simulink model "linear_model_GFM"  (R2018b)
settings: Solver=VariableStepAuto  StartTime=0.0  StopTime=0  RelTol=1e-3
InitFcn:
  | GFM_init
values from neighbouring files (symbols this model uses):
  Cf = Bf/w0    (= 6.36619772368e-05)    [MainTest.m]    (also in MainTest_v2.m)
  L = 1/Wbase    (= 0.00318309886184)    [Test.m]
  Pr = sym('Pr')    [MainTest.m]    (also in MainTest_v2.m)
  Qr = sym('Qr')    [MainTest.m]    (also in MainTest_v2.m)
  R = 1    [Test.m]
  Tm = 50*1e-3    (= 0.05)    [MainTest.m]    (also in MainTest_v2.m)
  w0 = 50*2*pi    (= 314.159265359)    [MainTest.m]    (also in MainTest_v2.m)
undefined symbols (not defined in the file or in its folder): Dp, Dq, I_d, I_LD, I_LQ, I_q, Ki, Kp, Tc, th, V, V_d, V_q, Vs
libraries: simulink x2
settings Model: Creator=balarko  LastModifiedBy=balarko
settings DataIOCC: ReturnWorkspaceOutputs=on

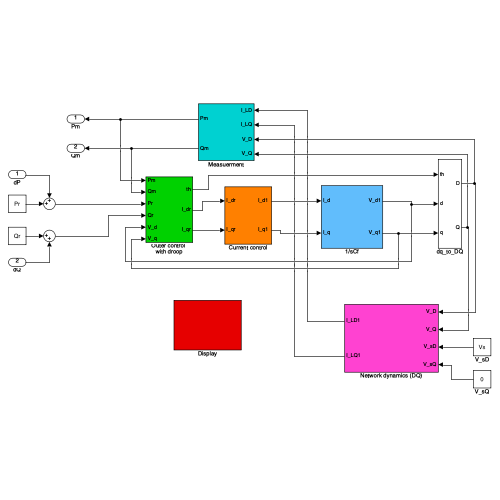
[thumbnail: Simulink's stored preview of the top-level diagram]
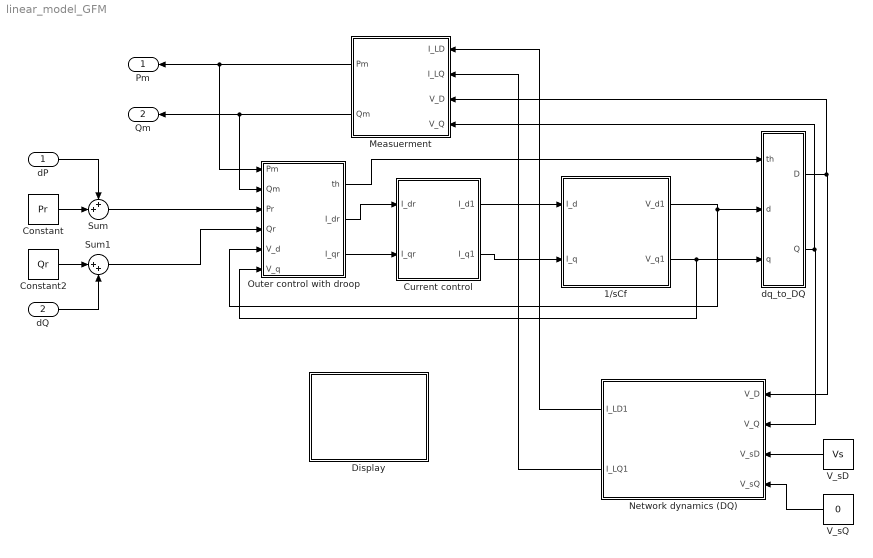
== system linear_model_GFM ==
  dP : Inport
  dQ : Inport  Port=2
  1/sCf : Subsystem
  Constant : Constant  Value=Pr
  Constant2 : Constant  Value=Qr
  Current control : Subsystem
  Display : Subsystem
  Measuerment : Subsystem
  Network dynamics (DQ) : Subsystem
  Outer control with droop : Subsystem
  Sum : Sum  Inputs=++|
  Sum1 : Sum  Inputs=|++
  V_sD : Constant  Value=Vs
  V_sQ : Constant  Value=0
  dq_to_DQ : Subsystem
  Pm : Outport
  Qm : Outport  Port=2
  wires:
  Outer control with droop/2(I_dr) -> Current control/1(I_dr)
  Outer control with droop/3(I_qr) -> Current control/2(I_qr)
  Current control/1("I_d1 ") -> 1/sCf/1(I_d)
  Current control/2("I_q1 ") -> 1/sCf/2(I_q)
  Network dynamics (DQ)/2(I_LQ1) -> Measuerment/2(I_LQ)
  1/sCf/1(V_d1) -> dq_to_DQ/2(d), Outer control with droop/5(V_d)
  1/sCf/2(V_q1) -> dq_to_DQ/3(q), Outer control with droop/6(V_q)
  V_sD/1 -> Network dynamics (DQ)/3(V_sD)
  V_sQ/1 -> Network dynamics (DQ)/4(V_sQ)
  Measuerment/2(Qm) -> Qm/1, Outer control with droop/2(Qm)
  Measuerment/1(Pm) -> Pm/1, Outer control with droop/1(Pm)
  Network dynamics (DQ)/1(I_LD1) -> Measuerment/1(I_LD)
  Sum/1 -> Outer control with droop/3(Pr)
  Constant/1 -> Sum/2
  Constant2/1 -> Sum1/1
  dQ/1 -> Sum1/2
  Sum1/1 -> Outer control with droop/4(Qr)
  dP/1 -> Sum/1
  dq_to_DQ/1(D) -> Measuerment/3(V_D), Network dynamics (DQ)/1(V_D)
  dq_to_DQ/2(Q) -> Measuerment/4(V_Q), Network dynamics (DQ)/2(V_Q)
  Outer control with droop/1(th) -> dq_to_DQ/1(th)

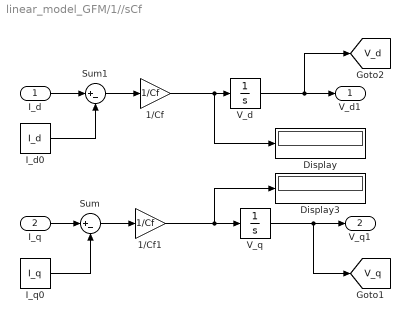
== system linear_model_GFM/1//sCf ==
  I_d : Inport
  I_q : Inport  Port=2
  1/Cf : Gain  Gain=1/Cf
  1/Cf1 : Gain  Gain=1/Cf
  Display : Display
  Display3 : Display
  I_d0 : Constant  Value=I_d
  I_q0 : Constant  Value=I_q
  Sum : Sum  Inputs=|+-
  Sum1 : Sum  Inputs=|+-
  V_d : Integrator  InitialCondition=V_d
  V_q : Integrator  InitialCondition=V_q
  V_d1 : Outport  VectorParamsAs1DForOutWhenUnconnected=off
  V_q1 : Outport  Port=2  VectorParamsAs1DForOutWhenUnconnected=off
  tag scope: V_d=global, V_q=global
  wires:
  V_d/1 -> [V_d], V_d1/1
  V_q/1 -> [V_q], V_q1/1
  1/Cf/1 -> Display/1, V_d/1
  1/Cf1/1 -> Display3/1, V_q/1
  I_q/1 -> Sum/1
  I_d/1 -> Sum1/1
  Sum1/1 -> 1/Cf/1
  I_d0/1 -> Sum1/2
  I_q0/1 -> Sum/2
  Sum/1 -> 1/Cf1/1

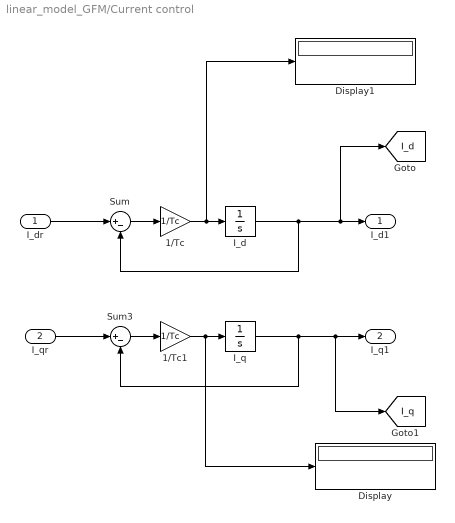
== system linear_model_GFM/Current control ==
  I_dr : Inport
  I_qr : Inport  Port=2
  1/Tc : Gain  Gain=1/Tc
  1/Tc1 : Gain  Gain=1/Tc
  Display : Display
  Display1 : Display
  "I_d " : Integrator  InitialCondition=I_d
  "I_q " : Integrator  InitialCondition=I_q
  Sum : Sum  Inputs=|+-
  Sum3 : Sum  Inputs=|+-
  "I_d1 " : Outport  VectorParamsAs1DForOutWhenUnconnected=off
  "I_q1 " : Outport  Port=2  VectorParamsAs1DForOutWhenUnconnected=off
  tag scope: I_d=global, I_q=global
  wires:
  Sum/1 -> 1/Tc/1
  1/Tc/1 -> Display1/1, "I_d "/1
  I_dr/1 -> Sum/1
  "I_d "/1 -> [I_d], "I_d1 "/1, Sum/2
  "I_q "/1 -> [I_q], "I_q1 "/1, Sum3/2
  Sum3/1 -> 1/Tc1/1
  1/Tc1/1 -> Display/1, "I_q "/1
  I_qr/1 -> Sum3/1

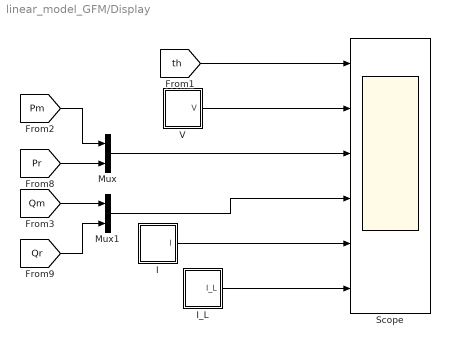
== system linear_model_GFM/Display ==
  I : Subsystem
  I_L : Subsystem
  Mux : Mux  Inputs=2
  Mux1 : Mux  Inputs=2
  Scope : Scope  NumInputPorts=6
  V : Subsystem
  wires:
  [Pr] -> Mux/2
  [Qm] -> Mux1/1
  [Qr] -> Mux1/2
  [Pm] -> Mux/1
  [th] -> Scope/1
  V/1(V) -> Scope/2
  Mux/1 -> Scope/3
  I_L/1(I_L) -> Scope/6
  I/1(I) -> Scope/5
  Mux1/1 -> Scope/4

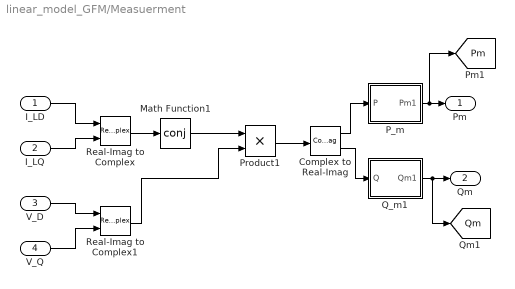
== system linear_model_GFM/Measuerment ==
  I_LD : Inport
  I_LQ : Inport  Port=2
  V_D : Inport  Port=3
  V_Q : Inport  Port=4
  Complex to Real-Imag : ComplexToRealImag
  Math Function1 : Math  Operator=conj  SaturateOnIntegerOverflow=on
  P_m : Subsystem
  Product1 : Product
  Q_m1 : Subsystem
  Real-Imag to Complex : RealImagToComplex
  Real-Imag to Complex1 : RealImagToComplex
  Pm : Outport  VectorParamsAs1DForOutWhenUnconnected=off
  Qm : Outport  Port=2  VectorParamsAs1DForOutWhenUnconnected=off
  tag scope: Pm=global, Qm=global
  wires:
  Real-Imag to Complex/1 -> Math Function1/1
  Math Function1/1 -> Product1/1
  Product1/1 -> Complex to Real-Imag/1
  Real-Imag to Complex1/1 -> Product1/2
  I_LD/1 -> Real-Imag to Complex/1
  I_LQ/1 -> Real-Imag to Complex/2
  V_D/1 -> Real-Imag to Complex1/1
  V_Q/1 -> Real-Imag to Complex1/2
  P_m/1(Pm1) -> [Pm], Pm/1
  Complex to Real-Imag/1 -> P_m/1(P)
  Complex to Real-Imag/2 -> Q_m1/1(Q)
  Q_m1/1(Qm1) -> [Qm], Qm/1

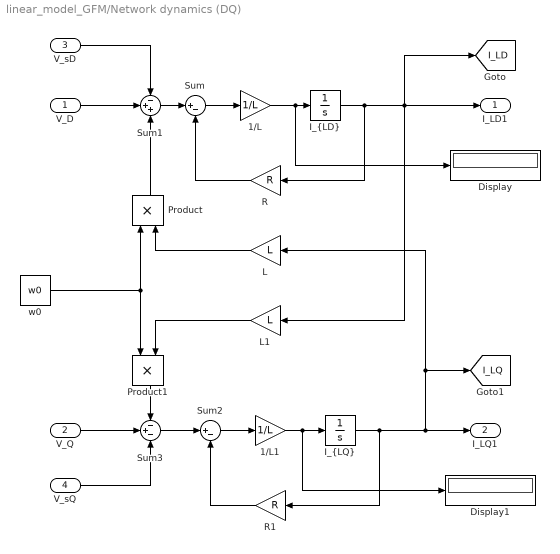
== system linear_model_GFM/Network dynamics (DQ) ==
  V_D : Inport
  V_Q : Inport  Port=2
  V_sD : Inport  Port=3
  V_sQ : Inport  Port=4
  1/L : Gain  Gain=1/L
  1/L1 : Gain  Gain=1/L
  Display : Display
  Display1 : Display
  "I_{LD}" : Integrator  InitialCondition=I_LD
  "I_{LQ}" : Integrator  InitialCondition=I_LQ
  L : Gain  Gain=L
  L1 : Gain  Gain=L
  Product : Product
  Product1 : Product
  R : Gain  Gain=R
  R1 : Gain  Gain=R
  Sum : Sum  Inputs=|+-
  Sum1 : Sum  Inputs=-++
  Sum2 : Sum  Inputs=|+-
  Sum3 : Sum  Inputs=-+-
  w0 : Constant  Value=w0
  I_LD1 : Outport  VectorParamsAs1DForOutWhenUnconnected=off
  I_LQ1 : Outport  Port=2  VectorParamsAs1DForOutWhenUnconnected=off
  tag scope: I_LD=global, I_LQ=global
  wires:
  Sum1/1 -> Sum/1
  V_sQ/1 -> Sum3/3
  1/L/1 -> Display/1, "I_{LD}"/1
  1/L1/1 -> Display1/1, "I_{LQ}"/1
  V_sD/1 -> Sum1/1
  Sum/1 -> 1/L/1
  "I_{LD}"/1 -> [I_LD], I_LD1/1, L1/1, R/1
  "I_{LQ}"/1 -> I_LQ1/1, [I_LQ], L/1, R1/1
  R/1 -> Sum/2
  Sum3/1 -> Sum2/1
  Sum2/1 -> 1/L1/1
  V_Q/1 -> Sum3/2
  R1/1 -> Sum2/2
  V_D/1 -> Sum1/2
  Product/1 -> Sum1/3
  Product1/1 -> Sum3/1
  w0/1 -> Product1/1, Product/1
  L/1 -> Product/2
  L1/1 -> Product1/2

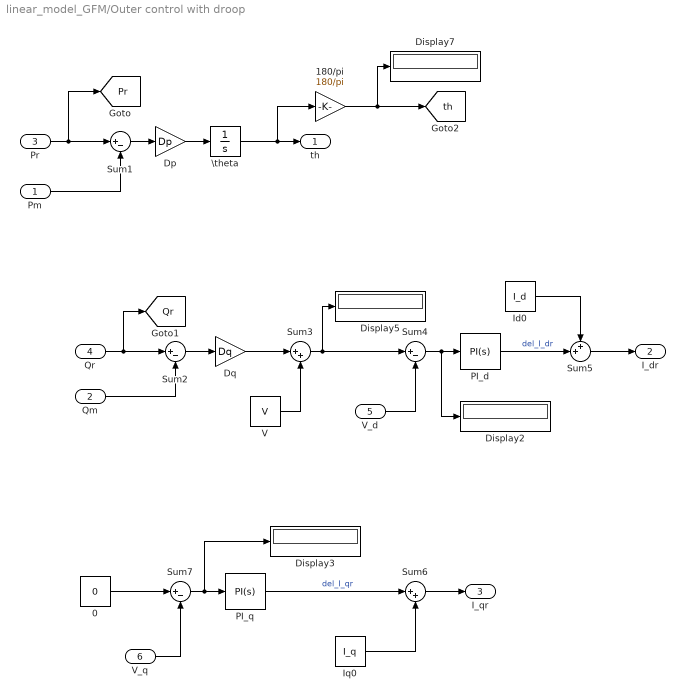
== system linear_model_GFM/Outer control with droop ==
  Pm : Inport
  Qm : Inport  Port=2
  Pr : Inport  Port=3
  Qr : Inport  Port=4
  V_d : Inport  Port=5
  V_q : Inport  Port=6
  0 : Constant  Value=0
  180/pi : Gain  Gain=180/pi
  Display{2..3,5,7} (4 alike) : Display
  Dp : Gain  Gain=Dp
  Dq : Gain  Gain=Dq
  Id0 : Constant  Value=I_d
  Iq0 : Constant  Value=I_q
  PI_d : simulink/Continuous/PID Controller  Controller=PI  Form=Parallel  TimeDomain=Continuous-time  SampleTime=-1  IntegratorMethod=Forward Euler  ControllerParametersSource=internal  P=Kp  I=Ki  D=0  N=100  UseFilter=on  TunerSelectOption=Transfer Function Based (PID Tuner App)  InitialConditionSource=internal  InitialConditionForIntegrator=0  InitialConditionForFilter=0  DifferentiatorICPrevScaledInput=0  ExternalReset=none  TrackingMode=off  Kt=1  LimitOutput=off  UpperSaturationLimit=inf  LowerSaturationLimit=-inf  LinearizeAsGain=on  AntiWindupMode=none  Kb=1  POutMin=[]  POutMax=[]  IOutMin=[]  IOutMax=[]  DOutMin=[]  DOutMax=[]  NOutMin=[]  NOutMax=[]  SumOutMin=[]  SumOutMax=[]  SaturationOutMin=[]  SaturationOutMax=[]  PParamMin=[]  PParamMax=[]  IParamMin=[]  IParamMax=[]  DParamMin=[]  DParamMax=[]  NParamMin=[]  NParamMax=[]  KbParamMin=[]  KbParamMax=[]  KtParamMin=[]  KtParamMax=[]  KbOutMin=[]  KbOutMax=[]  KtOutMin=[]  KtOutMax=[]  IntegratorOutMin=[]  IntegratorOutMax=[]  FilterOutMin=[]  FilterOutMax=[]  SumI1OutMin=[]  SumI1OutMax=[]  SumI2OutMin=[]  SumI2OutMax=[]  SumI3OutMin=[]  SumI3OutMax=[]  SumI4OutMin=[]  SumI4OutMax=[]  SumDOutMin=[]  SumDOutMax=[]  DifferentiatorOutMin=[]  DifferentiatorOutMax=[]  FilterDiffOutCoefMin=[]  FilterDiffOutCoefMax=[]  ReciprocalOutMin=[]  ReciprocalOutMax=[]  SumDenOutMin=[]  SumDenOutMax=[]  SumNumOutMin=[]  SumNumOutMax=[]  DivideOutMin=[]  DivideOutMax=[]  IntegratorContinuousStateAttributes='PI_d'  IntegratorStateMustResolveToSignalObject=off  IntegratorRTWStateStorageClass=Auto  FilterContinuousStateAttributes=''  FilterStateMustResolveToSignalObject=off  FilterRTWStateStorageClass=Auto  ParallelPVariant=InternalParameters  IdealPVariant=Disabled  IVariant=InternalParameters  DVariant=Disabled  IntegratorVariant=Continuous  SatVariant=Disabled  AWVariant=Passthrough  PCopyVariant=Disabled  TRVariant=Disabled  FdbkBlocksVariant=Forward  IdealPFdbkVariant=Disabled  SatFdbkVariant=Disabled  DerivativeFilterVariant=Disabled  NVariant=Disabled  NCopyVariant=Disabled_SignalSpec  FilterICVariant=Disabled  IntegratorICVariant=InternalICs  ExternalResetVariant=Disabled  TRSumVariant=Passthrough  SumFdbkVariant=Disabled  SumVariant=Sum_PI
  PI_q : simulink/Continuous/PID Controller  Controller=PI  Form=Parallel  TimeDomain=Continuous-time  SampleTime=-1  IntegratorMethod=Forward Euler  ControllerParametersSource=internal  P=Kp  I=Ki  D=0  N=100  UseFilter=on  TunerSelectOption=Transfer Function Based (PID Tuner App)  InitialConditionSource=internal  InitialConditionForIntegrator=0  InitialConditionForFilter=0  DifferentiatorICPrevScaledInput=0  ExternalReset=none  TrackingMode=off  Kt=1  LimitOutput=off  UpperSaturationLimit=inf  LowerSaturationLimit=-inf  LinearizeAsGain=on  AntiWindupMode=none  Kb=1  POutMin=[]  POutMax=[]  IOutMin=[]  IOutMax=[]  DOutMin=[]  DOutMax=[]  NOutMin=[]  NOutMax=[]  SumOutMin=[]  SumOutMax=[]  SaturationOutMin=[]  SaturationOutMax=[]  PParamMin=[]  PParamMax=[]  IParamMin=[]  IParamMax=[]  DParamMin=[]  DParamMax=[]  NParamMin=[]  NParamMax=[]  KbParamMin=[]  KbParamMax=[]  KtParamMin=[]  KtParamMax=[]  KbOutMin=[]  KbOutMax=[]  KtOutMin=[]  KtOutMax=[]  IntegratorOutMin=[]  IntegratorOutMax=[]  FilterOutMin=[]  FilterOutMax=[]  SumI1OutMin=[]  SumI1OutMax=[]  SumI2OutMin=[]  SumI2OutMax=[]  SumI3OutMin=[]  SumI3OutMax=[]  SumI4OutMin=[]  SumI4OutMax=[]  SumDOutMin=[]  SumDOutMax=[]  DifferentiatorOutMin=[]  DifferentiatorOutMax=[]  FilterDiffOutCoefMin=[]  FilterDiffOutCoefMax=[]  ReciprocalOutMin=[]  ReciprocalOutMax=[]  SumDenOutMin=[]  SumDenOutMax=[]  SumNumOutMin=[]  SumNumOutMax=[]  DivideOutMin=[]  DivideOutMax=[]  IntegratorContinuousStateAttributes='PI_q'  IntegratorStateMustResolveToSignalObject=off  IntegratorRTWStateStorageClass=Auto  FilterContinuousStateAttributes=''  FilterStateMustResolveToSignalObject=off  FilterRTWStateStorageClass=Auto  ParallelPVariant=InternalParameters  IdealPVariant=Disabled  IVariant=InternalParameters  DVariant=Disabled  IntegratorVariant=Continuous  SatVariant=Disabled  AWVariant=Passthrough  PCopyVariant=Disabled  TRVariant=Disabled  FdbkBlocksVariant=Forward  IdealPFdbkVariant=Disabled  SatFdbkVariant=Disabled  DerivativeFilterVariant=Disabled  NVariant=Disabled  NCopyVariant=Disabled_SignalSpec  FilterICVariant=Disabled  IntegratorICVariant=InternalICs  ExternalResetVariant=Disabled  TRSumVariant=Passthrough  SumFdbkVariant=Disabled  SumVariant=Sum_PI
  Sum{1..2,4,7} (4 alike) : Sum  Inputs=|+-
  Sum3 : Sum  Inputs=|++
  Sum5 : Sum  Inputs=++|
  Sum6 : Sum  Inputs=|++
  V : Constant  Value=V
  \theta : Integrator  InitialCondition=th*pi/180
  th : Outport
  I_dr : Outport  Port=2  VectorParamsAs1DForOutWhenUnconnected=off
  I_qr : Outport  Port=3  VectorParamsAs1DForOutWhenUnconnected=off
  tag scope: Pr=global, Qr=global, th=global
  wires:
  Pr/1 -> [Pr], Sum1/1
  Qm/1 -> Sum2/2
  Qr/1 -> [Qr], Sum2/1
  Pm/1 -> Sum1/2
  Sum1/1 -> Dp/1
  Sum2/1 -> Dq/1
  V/1 -> Sum3/2
  Sum4/1 -> Display2/1, PI_d/1
  Sum7/1 -> Display3/1, PI_q/1
  \theta/1 -> th/1, 180/pi/1
  Sum3/1 -> Sum4/1, Display5/1
  0/1 -> Sum7/1
  V_d/1 -> Sum4/2
  V_q/1 -> Sum7/2
  180/pi/1 -> Display7/1, [th]
  PI_d/1 -> Sum5/2  "del_I_dr"
  Sum5/1 -> I_dr/1
  PI_q/1 -> Sum6/1  "del_I_qr"
  Iq0/1 -> Sum6/2
  Id0/1 -> Sum5/1
  Sum6/1 -> I_qr/1
  Dp/1 -> \theta/1
  Dq/1 -> Sum3/1

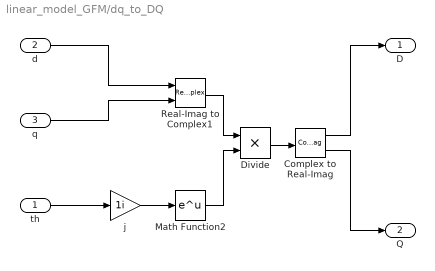
== system linear_model_GFM/dq_to_DQ ==
  th : Inport
  d : Inport  Port=2
  q : Inport  Port=3
  Complex to Real-Imag : ComplexToRealImag
  Divide : Product  Inputs=**
  Math Function2 : Math  SaturateOnIntegerOverflow=on
  Real-Imag to Complex1 : RealImagToComplex
  j : Gain  Gain=1i
  D : Outport  VectorParamsAs1DForOutWhenUnconnected=off
  Q : Outport  Port=2  VectorParamsAs1DForOutWhenUnconnected=off
  wires:
  Real-Imag to Complex1/1 -> Divide/1
  Complex to Real-Imag/2 -> Q/1
  j/1 -> Math Function2/1
  Math Function2/1 -> Divide/2
  d/1 -> Real-Imag to Complex1/1
  Complex to Real-Imag/1 -> D/1
  q/1 -> Real-Imag to Complex1/2
  Divide/1 -> Complex to Real-Imag/1
  th/1 -> j/1

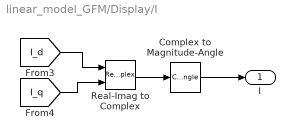
== system linear_model_GFM/Display/I ==
  Complex to Magnitude-Angle : ComplexToMagnitudeAngle  Output=Magnitude
  Real-Imag to Complex : RealImagToComplex
  I : Outport  VectorParamsAs1DForOutWhenUnconnected=off
  wires:
  [I_q] -> Real-Imag to Complex/2
  [I_d] -> Real-Imag to Complex/1
  Real-Imag to Complex/1 -> Complex to Magnitude-Angle/1
  Complex to Magnitude-Angle/1 -> I/1

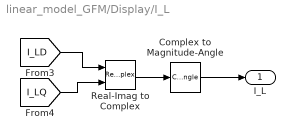
== system linear_model_GFM/Display/I_L ==
  Complex to Magnitude-Angle : ComplexToMagnitudeAngle  Output=Magnitude
  Real-Imag to Complex : RealImagToComplex
  I_L : Outport  VectorParamsAs1DForOutWhenUnconnected=off
  wires:
  [I_LQ] -> Real-Imag to Complex/2
  [I_LD] -> Real-Imag to Complex/1
  Real-Imag to Complex/1 -> Complex to Magnitude-Angle/1
  Complex to Magnitude-Angle/1 -> I_L/1

== system linear_model_GFM/Display/V ==
  Complex to Magnitude-Angle : ComplexToMagnitudeAngle  Output=Magnitude
  Real-Imag to Complex : RealImagToComplex
  V : Outport  VectorParamsAs1DForOutWhenUnconnected=off
  wires:
  [V_q] -> Real-Imag to Complex/2
  [V_d] -> Real-Imag to Complex/1
  Real-Imag to Complex/1 -> Complex to Magnitude-Angle/1
  Complex to Magnitude-Angle/1 -> V/1

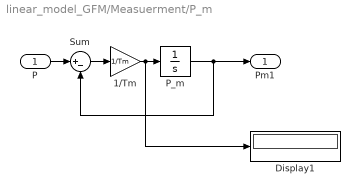
== system linear_model_GFM/Measuerment/P_m ==
  P : Inport
  1/Tm : Gain  Gain=1/Tm
  Display1 : Display
  P_m : Integrator  InitialCondition=Pr
  Sum : Sum  Inputs=|+-
  Pm1 : Outport  VectorParamsAs1DForOutWhenUnconnected=off
  wires:
  P/1 -> Sum/1
  Sum/1 -> 1/Tm/1
  1/Tm/1 -> Display1/1, P_m/1
  P_m/1 -> Sum/2, Pm1/1

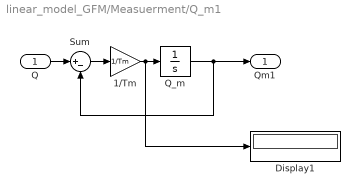
== system linear_model_GFM/Measuerment/Q_m1 ==
  Q : Inport
  1/Tm : Gain  Gain=1/Tm
  Display1 : Display
  Q_m : Integrator  InitialCondition=Qr
  Sum : Sum  Inputs=|+-
  Qm1 : Outport  VectorParamsAs1DForOutWhenUnconnected=off
  wires:
  Q/1 -> Sum/1
  Sum/1 -> 1/Tm/1
  1/Tm/1 -> Display1/1, Q_m/1
  Q_m/1 -> Sum/2, Qm1/1
